simulink model "ZSM_TeslaModelS_statKreisfahrt"  (R2020b)
settings: Solver=FixedStepDiscrete  StartTime=0.0  StopTime=simtime  FixedStep=stepsize  RelTol=1e-3
undefined symbols (not defined in the file): activate_stop, activate_stop_vmax, ay_stop, ayObs, ayStiff, Bat_param, deltav_ist, DiscIntNeverNeededParam, EG_wunsch, magnitude, mu_road_LF, mu_road_LR, mu_road_RF, mu_road_RR, par_ASR, par_MDT, par_TIR, par_VEH, select_delta_h, select_M_wheel, stepsize, t, temp_betriebsstrategie, temperature_LTrange, track_left, track_right
libraries: Library_ASK x36, simulink x16, pid_lib x2, dspstat3 x2, Library_Betriebsstrategie x2, vehicle_model x2, pacejka_trans x1
(part 2 of 7)

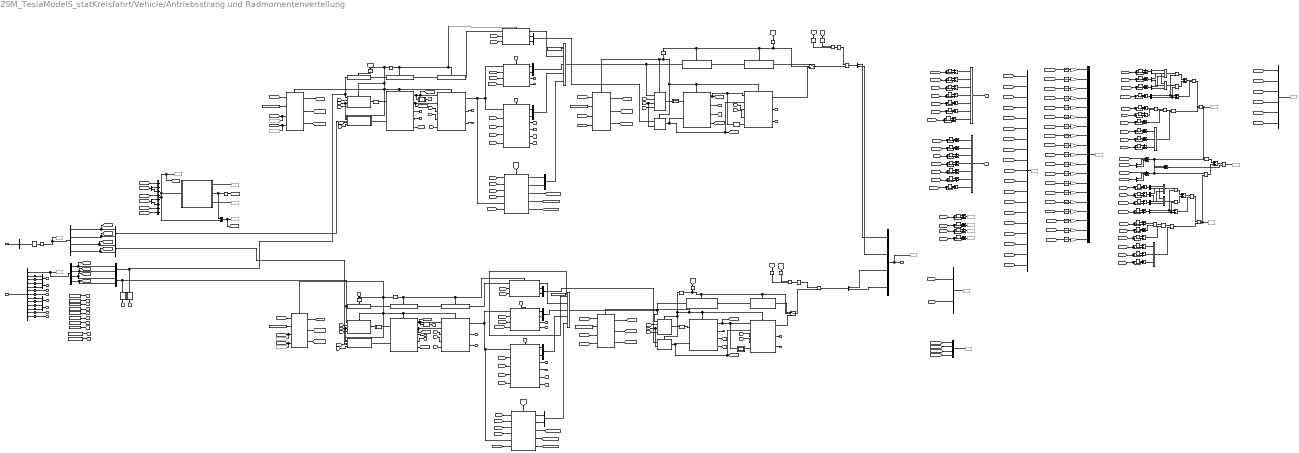
== system ZSM_TeslaModelS_statKreisfahrt/Vehicle/Antriebsstrang und Radmomentenverteilung ==
  note: Rekuperationsindex
  note: Rad-Wunsch-Momente
  note: Rad-Ist-Drehzahlen
  note: Vorderachse
  note: Hinterachse
  note: Overall efficiency of front and rear axle
  note: Gesamtwirkungsgrad des Antriebsstrangs EXKLUSIVE (ausgegraut) und INKLUSIVE (wenn nicht ausgegraut) E-Motor
  note: Verlustenergie
  note: Leistungsaufnahme der E-Maschinen
  note: Verlustleistungen
  note: einzelne Wirkungsgrade
  Ergebnisse der Betriebsstrategie : Inport
  Ergebnisse aus dem Fahrzeugmodell : Inport  Port=2
  Abs1 : Abs
  Add{,1..16,18..42,45..46} (44 alike) : Sum
  Add17 : Sum  Inputs=++++++++
  Add43 : Sum  Inputs=+++
  Add44 : Sum  Inputs=+++
  Batterie : Subsystem
  Bus Creator : BusCreator  Inputs=4
  Bus Creator1 : BusCreator  Inputs=2
  Bus Creator2 : BusCreator  Inputs=19
  Bus Creator3 : BusCreator  Inputs=19
  Bus Creator4 : BusCreator  Inputs=6
  Bus Creator5 : BusCreator  Inputs=4
  Bus Selector : BusSelector  OutputSignals=M_antr,Schaltstrategie.Übersetzungen.i_LF,Schaltstrategie.Übersetzungen.i_RF,Schaltstrategie.Übersetzungen.i_LR,Schaltstrategie.Übersetzungen.i_RR,Schaltstrategie.Übersetzungen.i_F,Schaltstrategie.Übersetzungen.i_R,Schaltstrategie.Wirkungsgrade.eta_LF,Schaltstrategie.Wirkungsgrade.eta_RF,Schaltstrategie.Wirkungsgrade.eta_LR,Schaltstrategie.Wirkungsgrade.eta_RR,Schaltstrategie.Wirkungsgrade.eta_F,Schaltstrategie.Wirkungsgrade.eta_R
  Bus Selector1 : BusSelector  OutputSignals=omega
  Bus to Vector2 : BusToVector
  Constant1 : Constant  Value=par_MDT.AUS.akt.az_VA
  Constant11 : Constant  Value=par_MDT.HA.em.U_RMS
  Constant12 : Constant  Value=par_MDT.HA.em.U_RMS
  Constant13 : Constant  Value=par_MDT.VA.em.U_RMS
  Constant14 : Constant  Value=par_MDT.AUS.akt.TS_VA
  Constant15 : Constant  Value=par_MDT.AUS.akt.TS_HA
  Constant2 : Constant  Value=par_MDT.AUS.akt.az_HA
  Constant22 : Constant  Value=par_MDT.AUS.switch.MVS_HA
  Constant24 : Constant  Value=par_MDT.AUS.switch.MVS_VA
  Constant3 : Constant  Value=par_MDT.AUS.akt.OD_VA
  Constant4 : Constant  Value=par_MDT.AUS.akt.OD_HA
  Constant5 : Constant  Value=par_MDT.AUS.akt.eTV_VA
  Constant6 : Constant  Value=par_MDT.AUS.akt.eTV_HA
  Constant7 : Constant  Value=par_MDT.AUS.akt.rn_VA
  Constant8 : Constant  Value=par_MDT.AUS.akt.rn_HA
  Constant9 : Constant  Value=par_MDT.HA.em.U_RMS
  Demux : Demux
  Demux{1..2,4..15} (14 alike) : Demux  Outputs=2
  Demux3 : Demux
  Discrete-Time Integrator{,1..18} (19 alike) : DiscreteIntegrator  SampleTime=stepsize  ICPrevOutput=DiscIntNeverNeededParam  ICPrevScaledInput=DiscIntNeverNeededParam
  Divide : Product  Inputs=*/
  Divide1 : Product  Inputs=*/
  Divide2 : Product  Inputs=*/
  Drehzahlrückführung az HA : Subsystem
  Drehzahlrückführung az VA : Subsystem
  Drehzahlrückführung rn HA fuer mmG : Library_ASK/Drehzahlrückführung rn fuer mmG  SystemSampleTime=-1  VariantActivationTime=update diagram  Latency=0  AutoFrameSizeCalculation=off
  Drehzahlrückführung rn VA fuer mmG : Library_ASK/Drehzahlrückführung rn fuer mmG  SystemSampleTime=-1  VariantActivationTime=update diagram  Latency=0  AutoFrameSizeCalculation=off
  Elektrisches Überlagerungsgetriebe HA : Library_ASK/Elektrisches Überlagerungsgetriebe HA  SystemSampleTime=-1  VariantActivationTime=update diagram  Latency=0  AutoFrameSizeCalculation=off
      link override Constant: Value=par_MDT.HA.trans.etv.i.i12_I
      link override Constant1: Value=par_MDT.HA.trans.etv.eta.eta12_III
      link override Constant10: Value=par_MDT.HA.trans.etv.eta.etaVTV_34
      link override Constant12: Value=par_MDT.HA.trans.etv.eta.eta12_I
      link override Constant13: Value=par_MDT.HA.trans.etv.eta.eta12_II
      link override Constant2: Value=par_MDT.HA.trans.etv.i.i12_II
      link override Constant3: Value=par_MDT.HA.trans.etv.i.i12_III
      link override Constant4: Value=par_MDT.HA.trans.etv.i.i12_IV
      link override Constant5: Value=par_MDT.HA.trans.etv.M_max_Steuer
      link override Constant6: Value=par_MDT.HA.trans.etv.i.iVTV_1
      link override Constant7: Value=par_MDT.HA.trans.etv.i.iVTV_2
      link override Constant8: Value=par_MDT.HA.trans.etv.eta.eta12_IV
      link override Constant9: Value=par_MDT.HA.trans.etv.eta.etaVTV_12
      link override Momentenkennlinie SEM/M_Antr: BreakpointsForDimension1=par_MDT.HA.trans.etv.Kennfelder.MaxMotorTrqCurve_w  Table=par_MDT.HA.trans.etv.Kennfelder.MaxMotorTrqCurve_M
      link override Momentenkennlinie SEM/M_Reku: BreakpointsForDimension1=par_MDT.HA.trans.etv.Kennfelder.MaxGeneratorTrqCurve_w  Table=par_MDT.HA.trans.etv.Kennfelder.MaxGeneratorTrqCurve_M
      link override eUELG Steuermaschine/Wirkungsgradkennfeld nach Pesce: BreakpointsForDimension1=par_MDT.HA.trans.etv.Kennfelder.MotorEffMap3D_w  BreakpointsForDimension2=par_MDT.HA.trans.etv.Kennfelder.MotorEffMap3D_M  Table=par_MDT.HA.trans.etv.Kennfelder.MotorEffMap3D
  Elektrisches Überlagerungsgetriebe VA : Library_ASK/Elektrisches Überlagerungsgetriebe VA  SystemSampleTime=-1  VariantActivationTime=update diagram  Latency=0  AutoFrameSizeCalculation=off
      link override Constant: Value=par_MDT.VA.trans.etv.i.i12_I
      link override Constant1: Value=par_MDT.VA.trans.etv.eta.eta12_III
      link override Constant10: Value=par_MDT.VA.trans.etv.eta.etaVTV_34
      link override Constant12: Value=par_MDT.VA.trans.etv.eta.eta12_I
      link override Constant13: Value=par_MDT.VA.trans.etv.eta.eta12_II
      link override Constant2: Value=par_MDT.VA.trans.etv.i.i12_II
      link override Constant3: Value=par_MDT.VA.trans.etv.i.i12_III
      link override Constant4: Value=par_MDT.VA.trans.etv.i.i12_IV
      link override Constant5: Value=par_MDT.VA.trans.etv.M_max_Steuer
      link override Constant6: Value=par_MDT.VA.trans.etv.i.iVTV_1
      link override Constant7: Value=par_MDT.VA.trans.etv.i.iVTV_2
      link override Constant8: Value=par_MDT.VA.trans.etv.eta.eta12_IV
      link override Constant9: Value=par_MDT.VA.trans.etv.eta.etaVTV_12
      link override Momentenkennlinie SEM/M_Antr: BreakpointsForDimension1=par_MDT.VA.trans.etv.Kennfelder.MaxMotorTrqCurve_w  Table=par_MDT.VA.trans.etv.Kennfelder.MaxMotorTrqCurve_M
      link override Momentenkennlinie SEM/M_Reku: BreakpointsForDimension1=par_MDT.VA.trans.etv.Kennfelder.MaxGeneratorTrqCurve_w  Table=par_MDT.VA.trans.etv.Kennfelder.MaxGeneratorTrqCurve_M
      link override eUELG Steuermaschine/Wirkungsgradkennfeld nach Pesce: BreakpointsForDimension1=par_MDT.VA.trans.etv.Kennfelder.MotorEffMap3D_w  BreakpointsForDimension2=par_MDT.VA.trans.etv.Kennfelder.MotorEffMap3D_M  Table=par_MDT.VA.trans.etv.Kennfelder.MotorEffMap3D
  HA : Product  Inputs=7
  HA_diff1 : Product  Inputs=3
  Kein Getriebe{,1..3} (4 alike) : Library_ASK/Kein Getriebe  SystemSampleTime=-1  VariantActivationTime=update diagram  Latency=0  AutoFrameSizeCalculation=off
  Kein MVS : Library_ASK/Kein MVS  SystemSampleTime=-1  VariantActivationTime=update diagram  Latency=0  AutoFrameSizeCalculation=off
  Kein MVS1 : Library_ASK/Kein MVS  SystemSampleTime=-1  VariantActivationTime=update diagram  Latency=0  AutoFrameSizeCalculation=off
  Keine E-Maschine : Library_ASK/Keine E-Maschine  SystemSampleTime=-1  VariantActivationTime=update diagram  Latency=0  AutoFrameSizeCalculation=off
  Keine E-Maschine radnah : Library_ASK/Keine E-Maschine  SystemSampleTime=-1  VariantActivationTime=update diagram  Latency=0  AutoFrameSizeCalculation=off
  Keine E-Maschine radnah1 : Library_ASK/Keine E-Maschine  SystemSampleTime=-1  VariantActivationTime=update diagram  Latency=0  AutoFrameSizeCalculation=off
  Keine E-Maschine1 : Library_ASK/Keine E-Maschine  SystemSampleTime=-1  VariantActivationTime=update diagram  Latency=0  AutoFrameSizeCalculation=off
  Keine Rückführung : Library_ASK/Keine Rückführung  SystemSampleTime=-1  VariantActivationTime=update diagram  Latency=0  AutoFrameSizeCalculation=off
  Keine Rückführung1 : Library_ASK/Keine Rückführung  SystemSampleTime=-1  VariantActivationTime=update diagram  Latency=0  AutoFrameSizeCalculation=off
  LF : Product  Inputs=3
  LF1 : Product  Inputs=3
  Leistungselektronik AZ HA : Library_ASK/Leistungselektronik  Efficiency_Map=par_MDT.HA.inv.efficiency_map.efficiency_map_LE  Current=par_MDT.HA.inv.current  Voltage=par_MDT.HA.inv.voltage  Powerfactor=par_MDT.HA.inv.powerfactor  Powerfactor_Map=par_MDT.HA.inv.Powerfactor_map  Torque=par_MDT.HA.inv.torque  Speed=par_MDT.HA.inv.speed
  Leistungselektronik AZ VA : Library_ASK/Leistungselektronik  Efficiency_Map=par_MDT.VA.inv.efficiency_map.efficiency_map_LE  Current=par_MDT.VA.inv.current  Voltage=par_MDT.VA.inv.voltage  Powerfactor=par_MDT.VA.inv.powerfactor  Powerfactor_Map=par_MDT.VA.inv.Powerfactor_map  Torque=par_MDT.VA.inv.torque  Speed=par_MDT.VA.inv.speed
  Leistungselektronik RN HA : Library_ASK/Leistungselektronik  Efficiency_Map=par_MDT.HA.inv.efficiency_map.efficiency_map_LE  Current=par_MDT.HA.inv.current  Voltage=par_MDT.HA.inv.voltage  Powerfactor=par_MDT.HA.inv.powerfactor  Powerfactor_Map=par_MDT.HA.inv.Powerfactor_map  Torque=par_MDT.HA.inv.torque  Speed=par_MDT.HA.inv.speed
  Leistungselektronik RN VA : Library_ASK/Leistungselektronik  Efficiency_Map=par_MDT.VA.inv.efficiency_map.efficiency_map_LE  Current=par_MDT.VA.inv.current  Voltage=par_MDT.VA.inv.voltage  Powerfactor=par_MDT.VA.inv.powerfactor  Powerfactor_Map=par_MDT.VA.inv.Powerfactor_map  Torque=par_MDT.VA.inv.torque  Speed=par_MDT.VA.inv.speed
  Logical Operator{,1..15,32..53} (38 alike) : Logic  Operator=NOT  Inputs=1  AllPortsSameDT=off  OutDataTypeStr=boolean
  Logical Operator{16..24,26..28,30..31} (14 alike) : Logic  Operator=NOT  AllPortsSameDT=off  OutDataTypeStr=boolean
  Logical Operator25 : Logic  AllPortsSameDT=off  OutDataTypeStr=boolean
  Logical Operator29 : Logic  AllPortsSameDT=off  OutDataTypeStr=boolean
  MATLAB Function : MATLAB Function  TreatAsAtomicUnit=on
  MATLAB Function1 : MATLAB Function  TreatAsAtomicUnit=on
  MATLAB Function2 : MATLAB Function  TreatAsAtomicUnit=on
  MATLAB Function3 : MATLAB Function  TreatAsAtomicUnit=on
  MATLAB Function4 : MATLAB Function  TreatAsAtomicUnit=on
  MATLAB Function5 : MATLAB Function  TreatAsAtomicUnit=on
  Mehrstufiges und mehrgängiges Getriebe az : Library_ASK/Mehrstufiges und mehrgängiges Getriebe  SystemSampleTime=-1  VariantActivationTime=update diagram  Latency=0  AutoFrameSizeCalculation=off
  Mehrstufiges und mehrgängiges Getriebe az1 : Library_ASK/Mehrstufiges und mehrgängiges Getriebe  SystemSampleTime=-1  VariantActivationTime=update diagram  Latency=0  AutoFrameSizeCalculation=off
  Mehrstufiges und mehrgängiges Getriebe rn : Library_ASK/Mehrstufiges und mehrgängiges Getriebe  SystemSampleTime=-1  VariantActivationTime=update diagram  Latency=0  AutoFrameSizeCalculation=off
  Mehrstufiges und mehrgängiges Getriebe rn1 : Library_ASK/Mehrstufiges und mehrgängiges Getriebe  SystemSampleTime=-1  VariantActivationTime=update diagram  Latency=0  AutoFrameSizeCalculation=off
  Memory{,2,6..15} (12 alike) : Memory  InitialCondition=10
  Memory1 : Memory
  Momentenrückführung HA fuer mmG : Library_ASK/Momentenrückführung fuer mmG  SystemSampleTime=-1  VariantActivationTime=update diagram  Latency=0  AutoFrameSizeCalculation=off
  Momentenrückführung HA fuer mmG3 : Library_ASK/Momentenrückführung fuer mmG  SystemSampleTime=-1  VariantActivationTime=update diagram  Latency=0  AutoFrameSizeCalculation=off
  Momentenrückführung VA fuer mmG : Library_ASK/Momentenrückführung fuer mmG  SystemSampleTime=-1  VariantActivationTime=update diagram  Latency=0  AutoFrameSizeCalculation=off
  Momentenrückführung VA fuer mmG1 : Library_ASK/Momentenrückführung fuer mmG  SystemSampleTime=-1  VariantActivationTime=update diagram  Latency=0  AutoFrameSizeCalculation=off
  Multiport Switch1 : MultiPortSwitch  Inputs=4
  Multiport Switch2 : MultiPortSwitch  Inputs=4
  Mux{,1..9,15..18,22..23} (16 alike) : Mux  Inputs=2
  Offenes Differential HA : Library_ASK/Offenes Differential  M_max=par_MDT.HA.em.M_max_achse  i_max=par_MDT.HA.trans.imax
      link override Constant2: Value=par_MDT.AUS.eta_Kegel
  Offenes Differential VA : Library_ASK/Offenes Differential  M_max=par_MDT.VA.em.M_max_achse  i_max=par_MDT.VA.trans.imax
      link override Constant2: Value=par_MDT.AUS.eta_Kegel
  PT_HA1 : Subsystem
  PT_HA2 : Subsystem
  PT_VA : Subsystem
  PT_VA1 : Subsystem
  Product{1..14} (14 alike) : Product
  RF : Product  Inputs=3
  RF1 : Product  Inputs=3
  Simple E-Maschine HA : Library_ASK/Simple E-Maschine  Mot_Mmax_Curve=par_MDT.HA.em.MaxMotorTrqCurve_M  Mot_nmax_Curve=par_MDT.HA.em.MaxMotorTrqCurve_w  Gen_Mmax_Curve=par_MDT.HA.em.MaxGeneratorTrqCurve_M  Gen_nmax_Curve=par_MDT.HA.em.MaxGeneratorTrqCurve_w  Mot_Pesce_Mat=par_MDT.HA.em.MotorEffMap3D  Mot_Pesce_y=par_MDT.HA.em.MotorEffMap3D_w  Mot_Pesce_z=par_MDT.HA.em.MotorEffMap3D_M  Gen_Pesce_Mat=par_MDT.HA.em.GeneratorEffMap3D  Gen_Pesce_y=par_MDT.HA.em.GeneratorEffMap3D_w  Gen_Pesce_z=par_MDT.HA.em.GeneratorEffMap3D_M
  Simple E-Maschine VA : Library_ASK/Simple E-Maschine  Mot_Mmax_Curve=par_MDT.VA.em.MaxMotorTrqCurve_M  Mot_nmax_Curve=par_MDT.VA.em.MaxMotorTrqCurve_w  Gen_Mmax_Curve=par_MDT.VA.em.MaxGeneratorTrqCurve_M  Gen_nmax_Curve=par_MDT.VA.em.MaxGeneratorTrqCurve_w  Mot_Pesce_Mat=par_MDT.VA.em.MotorEffMap3D  Mot_Pesce_y=par_MDT.VA.em.MotorEffMap3D_w  Mot_Pesce_z=par_MDT.VA.em.MotorEffMap3D_M  Gen_Pesce_Mat=par_MDT.VA.em.GeneratorEffMap3D  Gen_Pesce_y=par_MDT.VA.em.GeneratorEffMap3D_w  Gen_Pesce_z=par_MDT.VA.em.GeneratorEffMap3D_M
  Simple E-Maschine radnah : Library_ASK/Simple E-Maschine radnah  Mot_Mmax_Curve=par_MDT.VA.em.MaxMotorTrqCurve_M  Mot_nmax_Curve=par_MDT.VA.em.MaxMotorTrqCurve_w  Gen_Mmax_Curve=par_MDT.VA.em.MaxGeneratorTrqCurve_M  Gen_nmax_Curve=par_MDT.VA.em.MaxGeneratorTrqCurve_w  Mot_Pesce_Mat=par_MDT.VA.em.MotorEffMap3D  Mot_Pesce_y=par_MDT.VA.em.MotorEffMap3D_w  Mot_Pesce_z=par_MDT.VA.em.MotorEffMap3D_M  Gen_Pesce_Mat=par_MDT.VA.em.GeneratorEffMap3D  Gen_Pesce_y=par_MDT.VA.em.GeneratorEffMap3D_w  Gen_Pesce_z=par_MDT.VA.em.GeneratorEffMap3D_M
  Simple E-Maschine radnah1 : Library_ASK/Simple E-Maschine radnah  Mot_Mmax_Curve=par_MDT.HA.em.MaxMotorTrqCurve_M  Mot_nmax_Curve=par_MDT.HA.em.MaxMotorTrqCurve_w  Gen_Mmax_Curve=par_MDT.HA.em.MaxGeneratorTrqCurve_M  Gen_nmax_Curve=par_MDT.HA.em.MaxGeneratorTrqCurve_w  Mot_Pesce_Mat=par_MDT.HA.em.MotorEffMap3D  Mot_Pesce_y=par_MDT.HA.em.MotorEffMap3D_w  Mot_Pesce_z=par_MDT.HA.em.MotorEffMap3D_M  Gen_Pesce_Mat=par_MDT.HA.em.GeneratorEffMap3D  Gen_Pesce_y=par_MDT.HA.em.GeneratorEffMap3D_w  Gen_Pesce_z=par_MDT.HA.em.GeneratorEffMap3D_M
  Sum1 : Sum
  Switch1 : Switch  Criteria=u2 > Threshold
  Switch3 : Switch  Criteria=u2 > Threshold
  To Workspace : ToWorkspace  Commented=on  VariableName=n_Rad_ist  SampleTime=-1
      settings: Decimation=savedec  Save2DSignal=2-D array (concatenate along first dimension)
  To Workspace11 : ToWorkspace  Commented=on  VariableName=Batt_SOC  SaveFormat=Timeseries  SampleTime=-1
  To Workspace12 : ToWorkspace  Commented=on  VariableName=Batt_C_Rate  SaveFormat=Timeseries  SampleTime=-1
  To Workspace20 : ToWorkspace  Commented=on  VariableName=eta_ges  SaveFormat=Timeseries  SampleTime=-1
      settings: Decimation=savedec
  To Workspace3 : ToWorkspace  Commented=on  VariableName=P_Batt  SaveFormat=Timeseries  SampleTime=-1
  To Workspace4 : ToWorkspace  Commented=on  VariableName=M_antr  SaveFormat=Timeseries  SampleTime=-1
  To Workspace5 : ToWorkspace  Commented=on  VariableName=M_Rad_W  SampleTime=-1
      settings: Decimation=savedec  Save2DSignal=2-D array (concatenate along first dimension)
  To Workspace9 : ToWorkspace  Commented=on  VariableName=P_LE_DC  SaveFormat=Timeseries  SampleTime=-1
  To Ws 1 : ToWorkspace  Commented=on  VariableName=pv_ges  SaveFormat=Timeseries  SampleTime=-1
      settings: Decimation=savedec  Save2DSignal=2-D array (concatenate along first dimension)
  To Ws 10 : ToWorkspace  Commented=on  VariableName=eta_EM_rn_HA  SaveFormat=Timeseries  SampleTime=-1
      settings: Decimation=savedec  Save2DSignal=2-D array (concatenate along first dimension)
  To Ws 11 : ToWorkspace  Commented=on  VariableName=eta_LE  SaveFormat=Timeseries  SampleTime=-1
      settings: Decimation=savedec  Save2DSignal=2-D array (concatenate along first dimension)
  To Ws 12 : ToWorkspace  Commented=on  VariableName=eta_AS_ges  SaveFormat=Timeseries  SampleTime=-1
      settings: Decimation=savedec  Save2DSignal=2-D array (concatenate along first dimension)
  To Ws 14 : ToWorkspace  Commented=on  VariableName=sv_n_mot_az_ha  SaveFormat=Timeseries  SampleTime=-1
      settings: Decimation=savedec  Save2DSignal=2-D array (concatenate along first dimension)
  To Ws 15 : ToWorkspace  Commented=on  VariableName=sv_n_mot_az_va  SaveFormat=Timeseries  SampleTime=-1
      settings: Decimation=savedec  Save2DSignal=2-D array (concatenate along first dimension)
  To Ws 2 : ToWorkspace  Commented=on  VariableName=sv_m_mot_az_va  SaveFormat=Timeseries  SampleTime=-1
      settings: Decimation=savedec  Save2DSignal=2-D array (concatenate along first dimension)
  To Ws 3 : ToWorkspace  Commented=on  VariableName=eta_VA  SaveFormat=Timeseries  SampleTime=-1
      settings: Decimation=savedec  Save2DSignal=2-D array (concatenate along first dimension)
  To Ws 4 : ToWorkspace  Commented=on  VariableName=eta_HA  SaveFormat=Timeseries  SampleTime=-1
      settings: Decimation=savedec  Save2DSignal=2-D array (concatenate along first dimension)
  To Ws 5 : ToWorkspace  Commented=on  VariableName=Ev_ges  SaveFormat=Timeseries  SampleTime=-1
      settings: Decimation=savedec  Save2DSignal=2-D array (concatenate along first dimension)
  To Ws 6 : ToWorkspace  Commented=on  VariableName=P_el  SaveFormat=Timeseries  SampleTime=-1
      settings: Decimation=savedec  Save2DSignal=2-D array (concatenate along first dimension)
  To Ws 7 : ToWorkspace  Commented=on  VariableName=eta_EM_az_VA  SaveFormat=Timeseries  SampleTime=-1
      settings: Decimation=savedec  Save2DSignal=2-D array (concatenate along first dimension)
  To Ws 8 : ToWorkspace  Commented=on  VariableName=eta_EM_rn_VA  SaveFormat=Timeseries  SampleTime=-1
      settings: Decimation=savedec  Save2DSignal=2-D array (concatenate along first dimension)
  To Ws 9 : ToWorkspace  Commented=on  VariableName=eta_EM_az_HA  SaveFormat=Timeseries  SampleTime=-1
      settings: Decimation=savedec  Save2DSignal=2-D array (concatenate along first dimension)
  "To Ws 13 " : ToWorkspace  Commented=on  VariableName=sv_m_mot_az_ha  SaveFormat=Timeseries  SampleTime=-1
      settings: Decimation=savedec  Save2DSignal=2-D array (concatenate along first dimension)
  Torque Splitter v2 C. Angerer 10/1 : Library_ASK/Torque Splitter v2 C. Angerer 10//2018  SystemSampleTime=-1  VariantActivationTime=update diagram  Latency=0  AutoFrameSizeCalculation=off
  Torque Splitter v2 C. Angerer 10/2018 : Library_ASK/Torque Splitter v2 C. Angerer 10//2018  SystemSampleTime=-1  VariantActivationTime=update diagram  Latency=0  AutoFrameSizeCalculation=off
  VA : Product  Inputs=7
  VA_diff : Product  Inputs=3
  kWs --> kWh{,1..18} (19 alike) : Gain  Gain=1/3600
  w/o E-maschine HA : Product  Inputs=**
  w/o E-maschine VA : Product  Inputs=**
  M_antr : Outport  VectorParamsAs1DForOutWhenUnconnected=off
  wires:
  Bus Selector1/1 -> Bus to Vector2/1  "<omega>"
  Ergebnisse aus dem Fahrzeugmodell/1 -> Bus Selector1/1
  [OD_VA] -> Offenes Differential VA/Enable
  Mux/1 -> Keine Rückführung/1, Momentenrückführung VA fuer mmG/1, MATLAB Function/1(u)
  Demux/1 -> Mux/1, [M_Rad_W_RF]  "M_Rad_W_RF"
  Demux/2 -> Mux/2, [M_Rad_W_LF]  "M_Rad_W_LF"
  Logical Operator16/1 -> Kein MVS/Enable, Kein Getriebe/Enable, Keine E-Maschine/Enable
  Kein MVS/1 -> Multiport Switch1/2  "2"
  Demux/4 -> [M_Rad_W_LR], Mux1/2  "M_Rad_W_LR"
  Demux/3 -> Mux1/1, [M_Rad_W_RR]  "M_Rad_W_RR"
  Bus Creator/1 -> To Workspace4/1, M_antr/1
  Offenes Differential VA/2 -> Mux2/2  "1"
  Offenes Differential VA/1 -> Mux2/1  "1"
  Elektrisches Überlagerungsgetriebe VA/2 -> Mux3/2
  Elektrisches Überlagerungsgetriebe VA/1 -> Mux3/1
  Mux2/1 -> Multiport Switch1/3  "2"
  Demux1/1 -> Bus Creator/1  "M_antr_RF"
  Demux1/2 -> Bus Creator/2  "M_antr_LF"
  Kein Getriebe2/1 -> Switch3/1
  Constant24/1 -> Multiport Switch1/1
  [n_Rad_RF] -> Kein MVS/2
  [n_Rad_LF] -> Kein MVS/3
  Kein Getriebe/1 -> Kein MVS/1
  Mux15/1 -> Drehzahlrückführung az VA/3("Radrehzahlen ")
  Simple E-Maschine VA/3 -> [pv_simEM_az_VA]
  Kein MVS/2 -> Mux8/1
  Kein MVS/3 -> Mux8/2
  Demux3/1 -> Mux15/1, [n_Rad_RF]
  Demux3/2 -> Mux15/2, [n_Rad_LF]
  Demux3/3 -> Mux16/1, [n_Rad_RR]
  Demux3/4 -> [n_Rad_LR], Mux16/2
  Memory1/1 -> To Workspace/1, Demux3/1  "n_Rad_ist"
  Momentenrückführung VA fuer mmG/1 -> PT_VA1/1(M)
  Keine E-Maschine/1 -> Kein Getriebe/1
  Mux3/1 -> Multiport Switch1/4
  Multiport Switch1/1 -> Momentenrückführung VA fuer mmG1/1, Keine E-Maschine radnah/1  "2"
  Mux8/1 -> Drehzahlrückführung rn VA fuer mmG/1
  Keine E-Maschine radnah/1 -> Kein Getriebe2/1
  Demux2/1 -> Bus Creator/3  "M_antr_RR"
  Demux2/2 -> Bus Creator/4  "M_antr_LR"
  Bus to Vector2/1 -> Memory1/1
  Ergebnisse der Betriebsstrategie/1 -> Bus Selector/1
  Bus Selector/1 -> To Workspace5/1, Demux/1  "<M_antr>"
  [n_Rad_LF] -> Offenes Differential VA/3
  [n_Rad_RF] -> Elektrisches Überlagerungsgetriebe VA/2
  [n_Rad_LF] -> Elektrisches Überlagerungsgetriebe VA/3
  [M_Rad_W_RF] -> Elektrisches Überlagerungsgetriebe VA/4
  [M_Rad_W_LF] -> Elektrisches Überlagerungsgetriebe VA/5
  [n_Rad_RF] -> Offenes Differential VA/2
  [az_VA] -> Logical Operator16/1, Momentenrückführung VA fuer mmG/Enable, Mehrstufiges und mehrgängiges Getriebe az/Enable, Simple E-Maschine VA/Enable, Leistungselektronik AZ VA/Enable, Drehzahlrückführung az VA/1(Aktivator az), Logical Operator17/1
  Mehrstufiges und mehrgängiges Getriebe rn/1 -> Switch3/3
  [rn_VA] -> Logical Operator22/1
  [eta_VA] -> Momentenrückführung VA fuer mmG1/2
  [i_Gang_az_VA] -> Drehzahlrückführung az VA/2("i_Gang "), Momentenrückführung VA fuer mmG/3
  Keine Rückführung/1 -> Keine E-Maschine/1
  Mux17/1 -> [i_Gang_rn_VA]
  Mux18/1 -> [i_Gang_rn_HA]
  Mux22/1 -> [eta_Gang_rn_VA]
  Mux23/1 -> [eta_Gang_rn_HA]
  [i_Gang_rn_VA] -> Momentenrückführung VA fuer mmG1/3, Drehzahlrückführung rn VA fuer mmG/2
  [OD_HA] -> Offenes Differential HA/Enable
  [eTV_HA] -> Elektrisches Überlagerungsgetriebe HA/Enable
  Logical Operator20/1 -> Kein MVS1/Enable, Kein Getriebe1/Enable, Keine E-Maschine1/Enable
  Kein MVS1/1 -> Multiport Switch2/2  "2"
  Offenes Differential HA/2 -> Mux4/2  "1"
  Offenes Differential HA/1 -> Mux4/1  "1"
  Elektrisches Überlagerungsgetriebe HA/2 -> Mux5/2
  Elektrisches Überlagerungsgetriebe HA/1 -> Mux5/1
  Mux4/1 -> Multiport Switch2/3  "2"
  Kein Getriebe3/1 -> Switch1/1
  [rn_HA] -> Logical Operator26/1
  Constant22/1 -> Multiport Switch2/1
  [n_Rad_RR] -> Kein MVS1/2
  [n_Rad_LR] -> Kein MVS1/3
  Kein Getriebe1/1 -> Kein MVS1/1
  Kein MVS1/2 -> Mux6/1
  Kein MVS1/3 -> Mux6/2
  Momentenrückführung HA fuer mmG/1 -> PT_HA1/1(M)
  Keine E-Maschine1/1 -> Kein Getriebe1/1
  Mux5/1 -> Multiport Switch2/4
  Momentenrückführung HA fuer mmG3/1 -> PT_HA2/1(M)
  Multiport Switch2/1 -> Keine E-Maschine radnah1/1, Momentenrückführung HA fuer mmG3/1  "2"
  Mux6/1 -> Drehzahlrückführung rn HA fuer mmG/1
  Drehzahlrückführung rn HA fuer mmG/1 -> Simple E-Maschine radnah1/2, Mehrstufiges und mehrgängiges Getriebe rn1/2, [n_mot_rn_ha]
  Keine E-Maschine radnah1/1 -> Kein Getriebe3/1
  [n_Rad_LR] -> Offenes Differential HA/3
  [n_Rad_RR] -> Elektrisches Überlagerungsgetriebe HA/2
  [n_Rad_LR] -> Elektrisches Überlagerungsgetriebe HA/3
  [M_Rad_W_RR] -> Elektrisches Überlagerungsgetriebe HA/4
  [M_Rad_W_LR] -> Elektrisches Überlagerungsgetriebe HA/5
  Simple E-Maschine radnah1/3 -> [eta_EM_rn_HA]
  [n_Rad_RR] -> Offenes Differential HA/2
  [az_HA] -> Leistungselektronik AZ HA/Enable, Logical Operator20/1, Momentenrückführung HA fuer mmG/Enable, Drehzahlrückführung az HA/1(Aktivator az), Mehrstufiges und mehrgängiges Getriebe az1/Enable, Simple E-Maschine HA/Enable, Logical Operator18/1
  Mehrstufiges und mehrgängiges Getriebe rn1/1 -> Switch1/3
  Mehrstufiges und mehrgängiges Getriebe rn1/3 -> [eta_GTR_rn_HA]
  Logical Operator21/1 -> Leistungselektronik RN HA/Enable, Simple E-Maschine radnah1/Enable, Mehrstufiges und mehrgängiges Getriebe rn1/Enable, Drehzahlrückführung rn HA fuer mmG/Enable, Momentenrückführung HA fuer mmG3/Enable
  [eta_HA] -> Momentenrückführung HA fuer mmG/2
  [eta_HA] -> Momentenrückführung HA fuer mmG3/2
  [i_Gang_az_HA] -> Momentenrückführung HA fuer mmG/3, Drehzahlrückführung az HA/2("i_Gang ")
  Keine Rückführung1/1 -> Keine E-Maschine1/1
  Logical Operator18/1 -> Keine Rückführung1/Enable
  [i_Gang_az_HA] -> Mehrstufiges und mehrgängiges Getriebe az1/3
  [eta_Gang_az_HA] -> Mehrstufiges und mehrgängiges Getriebe az1/4
  [i_Gang_rn_HA] -> Momentenrückführung HA fuer mmG3/3, Drehzahlrückführung rn HA fuer mmG/2
  [i_Gang_rn_HA] -> Mehrstufiges und mehrgängiges Getriebe rn1/3
  [eta_Gang_rn_HA] -> Mehrstufiges und mehrgängiges Getriebe rn1/4
  Mux16/1 -> Drehzahlrückführung az HA/3("Radrehzahlen ")
  Bus Selector/2 -> Memory/1  "<i_LF>"
  Bus Selector/3 -> Memory2/1  "<i_RF>"
  Bus Selector/4 -> Memory6/1  "<i_LR>"
  Bus Selector/5 -> Memory7/1  "<i_RR>"
  Bus Selector/6 -> Memory8/1  "<i_F>"
  Bus Selector/7 -> Memory9/1  "<i_R>"
  Bus Selector/8 -> Memory10/1  "<eta_LF>"
  Bus Selector/9 -> Memory11/1  "<eta_RF>"
  Bus Selector/10 -> Memory12/1  "<eta_LR>"
  Bus Selector/11 -> Memory13/1  "<eta_RR>"
  Bus Selector/12 -> Memory14/1  "<eta_F>"
  Bus Selector/13 -> Memory15/1  "<eta_R>"
  Memory/1 -> Mux17/1
  Memory2/1 -> Mux17/2
  Memory6/1 -> Mux18/1
  Memory7/1 -> Mux18/2
  Memory8/1 -> [i_Gang_az_VA]
  Memory9/1 -> [i_Gang_az_HA]
  Memory10/1 -> Mux22/1
  Memory11/1 -> Mux22/2
  Memory12/1 -> Mux23/1
  Memory13/1 -> Mux23/2
  Memory14/1 -> [eta_Gang_az_VA]
  Memory15/1 -> [eta_Gang_az_HA]
  Constant1/1 -> [az_VA]
  Constant2/1 -> [az_HA]
  Constant3/1 -> [OD_VA]
  Constant4/1 -> [OD_HA]
  Constant5/1 -> [eTV_VA]
  Constant6/1 -> [eTV_HA]
  Logical Operator17/1 -> Keine Rückführung/Enable
  Logical Operator19/1 -> Mehrstufiges und mehrgängiges Getriebe rn/Enable, Simple E-Maschine radnah/Enable, Drehzahlrückführung rn VA fuer mmG/Enable, Leistungselektronik RN VA/Enable, Momentenrückführung VA fuer mmG1/Enable
  MATLAB Function1/1(RIX) -> [RIX_HA]
  MATLAB Function/1(RIX) -> [RIX_VA]
  [RIX_VA] -> Momentenrückführung VA fuer mmG/4
  [RIX_HA] -> Momentenrückführung HA fuer mmG/4
  [RIX_VA] -> Momentenrückführung VA fuer mmG1/4
  [RIX_HA] -> Momentenrückführung HA fuer mmG3/4
  Elektrisches Überlagerungsgetriebe VA/3 -> [pv_ges_eUELG_VA]
  Elektrisches Überlagerungsgetriebe VA/4 -> [M_Steuer_eUELG_VA]
  Elektrisches Überlagerungsgetriebe VA/5 -> [eta_eUELG_VA]
  Elektrisches Überlagerungsgetriebe VA/6 -> [P_Batt_eUELG_VA]
  Elektrisches Überlagerungsgetriebe HA/6 -> [P_Batt_eUELG_HA]
  Elektrisches Überlagerungsgetriebe HA/5 -> [eta_eUELG_HA]
  Elektrisches Überlagerungsgetriebe HA/4 -> [M_Steuer_eUELG_HA]
  Elektrisches Überlagerungsgetriebe HA/3 -> [pv_ges_eUELG_HA]
  Simple E-Maschine VA/4 -> [eta_EM_az_VA]
  Mehrstufiges und mehrgängiges Getriebe az/3 -> [eta_GTR_az_VA]
  Mehrstufiges und mehrgängiges Getriebe az/2 -> [pv_GTR_az_VA]
  Offenes Differential VA/4 -> [eta_OD_VA]
  Offenes Differential VA/3 -> [pv_OD_VA]
  Simple E-Maschine radnah/2 -> [pv_simEM_rn_VA]
  Simple E-Maschine radnah/3 -> [eta_EM_rn_VA]
  Mehrstufiges und mehrgängiges Getriebe rn/2 -> [pv_GTR_rn_VA]
  Mehrstufiges und mehrgängiges Getriebe rn/3 -> [eta_GTR_rn_VA]
  Simple E-Maschine HA/3 -> [pv_simEM_az_HA]
  Simple E-Maschine HA/4 -> [eta_EM_az_HA]
  Mehrstufiges und mehrgängiges Getriebe az1/2 -> [pv_GTR_az_HA]
  Mehrstufiges und mehrgängiges Getriebe az1/3 -> [eta_GTR_az_HA]
  Simple E-Maschine radnah1/2 -> [pv_simEM_rn_HA]
  Mehrstufiges und mehrgängiges Getriebe rn1/2 -> [pv_GTR_rn_HA]
  [RIX_VA_Delayed] -> Offenes Differential VA/4
  Offenes Differential HA/3 -> [pv_OD_HA]
  Offenes Differential HA/4 -> [eta_OD_HA]
  [RIX_VA_Delayed] -> Mehrstufiges und mehrgängiges Getriebe az/5
  [eta_Gang_az_VA] -> Mehrstufiges und mehrgängiges Getriebe az/4
  [i_Gang_az_VA] -> Mehrstufiges und mehrgängiges Getriebe az/3
  [i_Gang_rn_VA] -> Mehrstufiges und mehrgängiges Getriebe rn/3
  [eta_Gang_rn_VA] -> Mehrstufiges und mehrgängiges Getriebe rn/4
  MATLAB Function3/1(RIX) -> Mehrstufiges und mehrgängiges Getriebe rn/5
  Simple E-Maschine HA/2 -> [n_mot_az_ha], Mehrstufiges und mehrgängiges Getriebe az1/2
  [RIX_HA_Delayed] -> Mehrstufiges und mehrgängiges Getriebe az1/5
  Momentenrückführung VA fuer mmG1/1 -> PT_VA/1(M)  "2"
  [eta_VA] -> Momentenrückführung VA fuer mmG/2
  PT_VA/1(M_d) -> Simple E-Maschine radnah/1
  PT_VA1/1(M_d) -> Simple E-Maschine VA/1
  PT_HA1/1(M_d) -> Simple E-Maschine HA/1
  PT_HA2/1(M_d) -> Simple E-Maschine radnah1/1
  Simple E-Maschine VA/5 -> [P_el_EM_az_VA]
  Simple E-Maschine radnah/4 -> [P_el_EM_rn_VA]
  Simple E-Maschine radnah1/4 -> [P_el_EM_rn_HA]
  Simple E-Maschine HA/5 -> [P_el_EM_az_HA]
  Constant8/1 -> [rn_HA]
  Constant7/1 -> [rn_VA]
  Logical Operator22/1 -> Logical Operator19/1, Keine E-Maschine radnah/Enable, Kein Getriebe2/Enable, Switch3/2
  [rn_VA] -> Logical Operator24/1
  [az_VA] -> Logical Operator23/1
  Logical Operator23/1 -> Logical Operator25/2
  Logical Operator24/1 -> Logical Operator25/1
  Switch3/1 -> w/o E-maschine VA/2
  w/o E-maschine VA/1 -> Demux1/1
  Logical Operator26/1 -> Switch1/2, Kein Getriebe3/Enable, Keine E-Maschine radnah1/Enable, Logical Operator21/1
  Logical Operator27/1 -> Logical Operator29/2
  Logical Operator28/1 -> Logical Operator29/1
  [rn_HA] -> Logical Operator28/1
  [az_HA] -> Logical Operator27/1
  Switch1/1 -> w/o E-maschine HA/2
  w/o E-maschine HA/1 -> Demux2/1
  Logical Operator29/1 -> Logical Operator30/1
  Logical Operator30/1 -> w/o E-maschine HA/1
  Logical Operator25/1 -> Logical Operator31/1
  Logical Operator31/1 -> w/o E-maschine VA/1
  [P_LE_DC_HA_RN] -> Demux6/1
  [P_LE_DC_VA_AZ] -> Add17/1
  Demux6/2 -> Add17/6
  Batterie/3(C-Rate) -> To Workspace12/1
  Add17/1 -> Batterie/1(P_LE_DC), [P_LE_DC], To Workspace9/1, Sum1/2
  Sum1/1 -> [P_Batt], To Workspace3/1
  Batterie/2(pv_batt) -> Sum1/1, Abs1/1
  Demux5/2 -> Add17/3
  Demux5/1 -> Add17/2
  Batterie/1(SOC) -> To Workspace11/1
  Abs1/1 -> [pv_Batt]
  [P_LE_DC_HA_AZ] -> Add17/4
  Demux6/1 -> Add17/5
  [P_LE_DC_VA_RN] -> Demux5/1
  [P_el_EM_rn_VA] -> Leistungselektronik RN VA/1
  Constant9/1 -> Leistungselektronik RN VA/2
  [m_mot_rn_va] -> Leistungselektronik RN VA/3
  [n_mot_rn_va] -> Leistungselektronik RN VA/4
  [P_el_EM_rn_HA] -> Leistungselektronik RN HA/1
  Constant11/1 -> Leistungselektronik RN HA/2
  [m_mot_rn_ha] -> Leistungselektronik RN HA/3
  [n_mot_rn_ha] -> Leistungselektronik RN HA/4
  [P_el_EM_az_HA] -> Leistungselektronik AZ HA/1
  Constant12/1 -> Leistungselektronik AZ HA/2
  [m_mot_az_ha] -> "To Ws 13 "/1, Leistungselektronik AZ HA/3
  [n_mot_az_ha] -> To Ws 14/1, Leistungselektronik AZ HA/4
  [P_el_EM_az_VA] -> Leistungselektronik AZ VA/1
  Constant13/1 -> Leistungselektronik AZ VA/2
  [m_mot_az_va] -> To Ws 2/1, Leistungselektronik AZ VA/3
  [n_mot_az_va] -> To Ws 15/1, Leistungselektronik AZ VA/4
  Leistungselektronik AZ VA/1 -> [eta_LE_VA_AZ]
  Leistungselektronik AZ VA/2 -> [pv_LE_VA_AZ]
  Leistungselektronik AZ VA/3 -> [P_LE_DC_VA_AZ]
  Leistungselektronik AZ HA/1 -> [eta_LE_HA_AZ]
  Leistungselektronik AZ HA/2 -> [pv_LE_HA_AZ]
  Leistungselektronik AZ HA/3 -> [P_LE_DC_HA_AZ]
  Leistungselektronik RN HA/1 -> [eta_LE_HA_RN]
  Leistungselektronik RN HA/2 -> [pv_LE_HA_RN]
  Leistungselektronik RN HA/3 -> [P_LE_DC_HA_RN]
  Leistungselektronik RN VA/1 -> [eta_LE_VA_RN]
  Leistungselektronik RN VA/2 -> [pv_LE_VA_RN]
  Leistungselektronik RN VA/3 -> [P_LE_DC_VA_RN]
  Mehrstufiges und mehrgängiges Getriebe az1/1 -> Offenes Differential HA/1, Torque Splitter v2 C. Angerer 10/1/5, Elektrisches Überlagerungsgetriebe HA/1
  [TS_HA] -> Torque Splitter v2 C. Angerer 10/1/Enable
  Constant15/1 -> [TS_HA]
  Constant14/1 -> [TS_VA]
  Torque Splitter v2 C. Angerer 10/1/3 -> [n_Kupplung_geschlossen_HA]
  Torque Splitter v2 C. Angerer 10/1/2 -> Mux7/2
  Torque Splitter v2 C. Angerer 10/1/1 -> Mux7/1
  Torque Splitter v2 C. Angerer 10/1/4 -> [p_v_TS_HA]
  Torque Splitter v2 C. Angerer 10/1/5 -> [eta_TS_HA]
  [RIX_HA_Delayed] -> Torque Splitter v2 C. Angerer 10/1/6
  [M_Rad_W_LR] -> Torque Splitter v2 C. Angerer 10/1/4
  [M_Rad_W_RR] -> Torque Splitter v2 C. Angerer 10/1/3
  [n_Rad_LR] -> Torque Splitter v2 C. Angerer 10/1/2
  [n_Rad_RR] -> Torque Splitter v2 C. Angerer 10/1/1
  Mehrstufiges und mehrgängiges Getriebe az/1 -> Torque Splitter v2 C. Angerer 10/2018/5, Offenes Differential VA/1, Elektrisches Überlagerungsgetriebe VA/1
  Mux9/1 -> Multiport Switch1/5
  Torque Splitter v2 C. Angerer 10/2018/5 -> [eta_TS_VA]
  Torque Splitter v2 C. Angerer 10/2018/1 -> Mux9/1
  Torque Splitter v2 C. Angerer 10/2018/2 -> Mux9/2
  Torque Splitter v2 C. Angerer 10/2018/3 -> [n_Kupplung_geschlossen_VA]
  Torque Splitter v2 C. Angerer 10/2018/4 -> [p_v_TS_VA]
  [M_Rad_W_RF] -> Torque Splitter v2 C. Angerer 10/2018/3
  [M_Rad_W_LF] -> Torque Splitter v2 C. Angerer 10/2018/4
  [n_Rad_RF] -> Torque Splitter v2 C. Angerer 10/2018/1
  [n_Rad_LF] -> Torque Splitter v2 C. Angerer 10/2018/2
  [TS_HA] -> Drehzahlrückführung az HA/5(TS_HA)
  [n_Kupplung_geschlossen_HA] -> Drehzahlrückführung az HA/4(n_Kupplung_geschlossen_HA)
  Drehzahlrückführung az HA/1(n_motor) -> Simple E-Maschine HA/2
  [n_Kupplung_geschlossen_VA] -> Drehzahlrückführung az VA/4(n_Kupplung_geschlossen_VA)
  [TS_VA] -> Drehzahlrückführung az VA/5(TS_VA)
  Drehzahlrückführung az VA/1(n_motor) -> Simple E-Maschine VA/2
  [P_el_EM_rn_HA] -> Bus Creator4/4  "P_el_EM_rn_HA"
  Logical Operator/1 -> Add/1
  Discrete-Time Integrator6/1 -> kWs --> kWh6/1
  [pv_simEM_az_HA] -> Bus Creator3/2  "pv_simEM_az_HA"
  Bus Creator2/1 -> To Ws 5/1
  [pv_LE_HA_AZ] -> Discrete-Time Integrator14/1  "pv_LE_HA_AZ"
  [pv_OD_HA] -> Discrete-Time Integrator5/1  "pv_OD_HA"
  kWs --> kWh5/1 -> Bus Creator2/6  "Ev_OD_HA"
  Discrete-Time Integrator5/1 -> kWs --> kWh5/1
  kWs --> kWh3/1 -> Bus Creator2/4  "Ev_GTR_az_HA"
  kWs --> kWh14/1 -> Bus Creator2/15  "Ev_LE_HA_AZ"
  [pv_OD_HA] -> Bus Creator3/6  "pv_OD_HA"
  [pv_simEM_rn_HA] -> Bus Creator3/10  "pv_simEM_rn_HA"
  [pv_simEM_rn_HA] -> Discrete-Time Integrator9/1  "pv_simEM_rn_HA"
  [pv_LE_HA_AZ] -> Bus Creator3/15  "pv_LE_HA_AZ"
  [pv_GTR_az_HA] -> Bus Creator3/4  "pv_simGTR_az_HA"
  Discrete-Time Integrator11/1 -> kWs --> kWh11/1
  Discrete-Time Integrator/1 -> kWs --> kWh/1
  [pv_GTR_rn_HA] -> Bus Creator3/12  "pv_simGTR_rn_HA"
  [eta_LE_VA_RN] -> Bus Creator5/2  "eta_LE_VA_RN"
  Bus Creator4/1 -> To Ws 6/1  "P_el_EM"
  [p_v_TS_VA] -> Discrete-Time Integrator17/1  "PV_TS_VA"
  kWs --> kWh17/1 -> Bus Creator2/18
  Add21/1 -> Demux4/1
  Add/1 -> To Ws 7/1
  [eta_EM_rn_HA] -> Logical Operator45/1, Add33/2
  Add37/1 -> Demux12/1
  Add40/1 -> Demux13/1
  kWs --> kWh11/1 -> Bus Creator2/12  "Ev_GTR_rn_HA"
  [eta_LE_HA_AZ] -> Bus Creator5/3  "eta_LE_HA_AZ"
  Demux9/2 -> Product5/2, Add29/2  "P_LF"
  Demux8/1 -> RF/1  "LE_RF"
  [P_LE_DC_VA_AZ] -> Add43/1
  Logical Operator48/1 -> Add35/1
  [p_v_TS_VA] -> Bus Creator3/18
  [eta_OD_VA] -> Bus Creator1/1  "eta_OD_VA"
  LF1/1 -> Product11/1
  [P_el_EM_az_HA] -> Bus Creator4/3  "P_el_EM_az_HA"
  Bus Creator3/1 -> To Ws 1/1  "pv_ges"
  [eta_eUELG_HA] -> Add35/2, Logical Operator48/1
  Discrete-Time Integrator7/1 -> kWs --> kWh7/1
  Add36/1 -> Product8/2
  [eta_EM_az_HA] -> Logical Operator51/1, Add38/2
  Add29/1 -> Divide/2
  Logical Operator45/1 -> Add33/1
  Logical Operator6/1 -> Add7/1
  Logical Operator4/1 -> Add5/1
  Logical Operator1/1 -> Add2/1
  Bus Creator1/1 -> To Workspace20/1
  [eta_2GTR_az_HA] -> Logical Operator10/1, Add11/2
  Add13/1 -> HA/4
  Product1/1 -> Product2/1  "EM"
  Logical Operator52/1 -> Add39/1
  [eta_EM_rn_VA] -> Logical Operator35/1, Add21/2
  [eta_LE_VA_AZ] -> Bus Creator5/1  "eta_LE_VA_AZ"
  Logical Operator34/1 -> Add20/1
  Demux7/2 -> LF/3  "GTR_LF"
  Demux4/2 -> LF/2  "EM_LF"
  [P_el_EM_az_VA] -> Bus Creator4/1  "P_el_EM_az_VA"
  Demux4/1 -> RF/2  "EM_RF"
  Logical Operator11/1 -> Add12/1
  kWs --> kWh13/1 -> Bus Creator2/14  "Ev_LE_VA_RN"
  [eta_TS_VA] -> Add19/2, Logical Operator37/1
  [eta_OD_VA] -> Logical Operator36/1, Add22/2
  Logical Operator39/1 -> Add24/1
  Logical Operator36/1 -> Add22/1
  kWs --> kWh9/1 -> Bus Creator2/10  "Ev_EM_rn_HA"
  [eta_eUELG_VA] -> Add5/2, Logical Operator4/1
  Add27/1 -> Product1/1  "LE"
  Logical Operator2/1 -> Add3/1
  Add15/1 -> HA/5
  [eta_GTR_rn_HA] -> Add15/2, Logical Operator14/1
  [eta_2GTR_rn_VA] -> Add8/2, Logical Operator7/1
  Discrete-Time Integrator4/1 -> kWs --> kWh4/1
  Logical Operator3/1 -> Add4/1
  kWs --> kWh18/1 -> Bus Creator2/19
  [eta_2GTR_az_VA] -> Add3/2, Logical Operator2/1
  Add5/1 -> VA/4
  Add10/1 -> HA/1
  Add6/1 -> To Ws 8/1
  Add22/1 -> VA_diff/1
  [p_v_TS_HA] -> Bus Creator3/19
  Product9/1 -> Product12/2  "HA"
  [eta_LE_VA_AZ] -> Logical Operator42/1, Add27/2
  Add43/1 -> Product13/2, Add45/1  "P_VA"
  [eta_eUELG_VA] -> Add23/2, Logical Operator38/1
  RF1/1 -> Product10/1
  [pv_simEM_az_VA] -> Bus Creator3/1  "pv_simEM_az_VA"
  Demux14/2 -> Add43/3
  Logical Operator38/1 -> Add23/1
  [pv_ges_eUELG_HA] -> Bus Creator3/8  "pv_eUELG_HA"
  [pv_simEM_rn_VA] -> Bus Creator3/9  "pv_simEM_rn_VA"
  VA/1 -> [eta_VA]
  [eta_OD_HA] -> Logical Operator46/1, Add34/2
  [eta_OD_VA] -> Logical Operator3/1, Add4/2
  [pv_OD_VA] -> Bus Creator3/5  "pv_OD_VA"
  Divide2/1 -> To Ws 12/1  "eta_AS_ges"
  Logical Operator12/1 -> Add13/1
  Add45/1 -> Divide2/2  "P_ges"
  [eta_EM_rn_VA] -> Logical Operator5/1, Add6/2
  [eta_EM_az_HA] -> Add9/2, Logical Operator8/1
  Discrete-Time Integrator12/1 -> kWs --> kWh12/1
  Add46/1 -> Divide2/1
  Product8/1 -> Product9/1  "GTR"
  Discrete-Time Integrator1/1 -> kWs --> kWh1/1
  Add16/1 -> HA/6
  Demux15/2 -> Add44/3
  Product10/1 -> Add42/1
  Add26/1 -> Product1/2
  Product12/1 -> To Ws 4/1, Product14/2  "eta_HA"
  Demux9/1 -> Add29/1, Product4/2  "P_RF"
  Bus Creator5/1 -> To Ws 11/1
  [eta_GTR_rn_VA] -> Logical Operator34/1, Add20/2
  Product14/1 -> Add46/2
  [pv_GTR_rn_VA] -> Bus Creator3/11  "pv_simGTR_rn_VA"
  [pv_ges_eUELG_VA] -> Discrete-Time Integrator6/1  "pv_eUELG_VA"
  Add35/1 -> HA_diff1/2
  [pv_GTR_rn_HA] -> Discrete-Time Integrator11/1  "pv_simGTR_rn_HA"
  [eta_GTR_az_HA] -> Logical Operator49/1, Add36/2
  Add14/1 -> To Ws 10/1
  Discrete-Time Integrator14/1 -> kWs --> kWh14/1
  VA_diff/1 -> Product3/2
  Demux10/1 -> RF1/2  "EM_RF"
  Product2/1 -> Product3/1  "GTR"
  [eta_OD_HA] -> Bus Creator1/2  "eta_OD_HA"
  [pv_GTR_az_VA] -> Discrete-Time Integrator2/1  "pv_simGTR_az_VA"
  [pv_GTR_az_HA] -> Discrete-Time Integrator3/1  "pv_simGTR_az_HA"
  [eta_EM_az_VA] -> Logical Operator41/1, Add26/2
  Demux15/1 -> Add44/2
  [pv_ges_eUELG_HA] -> Discrete-Time Integrator7/1  "pv_eUELG_HA"
  Add1/1 -> HA/7
  kWs --> kWh1/1 -> Bus Creator2/2  "Ev_EM_az_HA"
  Discrete-Time Integrator2/1 -> kWs --> kWh2/1
  Logical Operator50/1 -> Add37/1
  [eta_LE_HA_AZ] -> Logical Operator52/1, Add39/2
  kWs --> kWh10/1 -> Bus Creator2/11  "Ev_GTR_rn_VA"
  Logical Operator37/1 -> Add19/1
  Demux11/1 -> RF1/3  "GTR_RF"
  Add39/1 -> Product7/1  "LE"
  Discrete-Time Integrator3/1 -> kWs --> kWh3/1
  [P_LE_DC_HA_RN] -> Demux15/1
  Demux7/1 -> RF/3  "GTR_RF"
  RF/1 -> Product4/1
  Demux14/1 -> Add43/2
  Discrete-Time Integrator17/1 -> kWs --> kWh17/1
  Logical Operator15/1 -> Add16/1
  Logical Operator49/1 -> Add36/1
  Logical Operator9/1 -> Add10/1
  Discrete-Time Integrator8/1 -> kWs --> kWh8/1
  [eta_LE_HA_RN] -> Bus Creator5/4  "eta_LE_HA_RN"
  kWs --> kWh15/1 -> Bus Creator2/16  "Ev_LE_HA_RN"
  [P_Batt] -> Bus Creator4/6  "pv_LE_VA_RN"
  Add20/1 -> Demux7/1
  [pv_GTR_rn_VA] -> Discrete-Time Integrator10/1  "pv_simGTR_rn_VA"
  Product11/1 -> Add42/2
  Add33/1 -> Demux10/1
  Logical Operator40/1 -> Add25/1
  Add32/1 -> Demux11/1
  Add34/1 -> HA_diff1/1
  Add38/1 -> Product7/2
  Logical Operator14/1 -> Add15/1
  Divide/1 -> Product6/1
  Add31/1 -> HA_diff1/3
  Logical Operator5/1 -> Add6/1
  [pv_simEM_az_HA] -> Discrete-Time Integrator1/1  "pv_simEM_az_HA"
  [pv_GTR_az_VA] -> Bus Creator3/3  "pv_simGTR_az_VA"
  Demux12/2 -> LF1/1  "LE_LF"
  Demux13/2 -> Product11/2, Add41/2  "P_LF"
  kWs --> kWh6/1 -> Bus Creator2/7  "Ev_eUELG_VA"
  [eta_TS_HA] -> Add31/2, Logical Operator47/1
  Add41/1 -> Divide1/2
  Demux13/1 -> Add41/1, Product10/2  "P_RF"
  Product6/1 -> To Ws 3/1, Product13/1  "eta_VA"
  Add42/1 -> Divide1/1
  Logical Operator46/1 -> Add34/1
  [P_LE_DC_HA_AZ] -> Add44/1
  [pv_LE_VA_RN] -> Bus Creator3/14  "pv_LE_VA_RN"
  Discrete-Time Integrator13/1 -> kWs --> kWh13/1
  [eta_TS_VA] -> Add18/2, Logical Operator33/1
  Add9/1 -> To Ws 9/1
  Add18/1 -> VA/7
  [eta_TS_HA] -> Add1/2, Logical Operator32/1
  [eta_LE_HA_RN] -> Add37/2, Logical Operator50/1
  Logical Operator32/1 -> Add1/1
  Add3/1 -> VA/2
  kWs --> kWh2/1 -> Bus Creator2/3  "Ev_GTR_az_VA"
  [P_LE_DC] -> Bus Creator4/5  "pv_LE_VA_AZ"
  [p_v_TS_HA] -> Discrete-Time Integrator18/1  "PV_TS_HA"
  Discrete-Time Integrator18/1 -> kWs --> kWh18/1
  Add11/1 -> HA/2
  Logical Operator44/1 -> Add32/1
  Add12/1 -> HA/3
  [eta_2GTR_rn_HA] -> Logical Operator15/1, Add16/2
  [P_LE_DC_VA_RN] -> Demux14/1
  Discrete-Time Integrator15/1 -> kWs --> kWh15/1
  [eta_EM_rn_HA] -> Add14/2, Logical Operator13/1
  Add4/1 -> VA/3
  Add8/1 -> VA/6
  Logical Operator8/1 -> Add9/1
  [eta_eUELG_HA] -> Logical Operator12/1, Add13/2
  Discrete-Time Integrator10/1 -> kWs --> kWh10/1
  [eta_OD_HA] -> Add12/2, Logical Operator11/1
  Add2/1 -> VA/1
  [pv_simEM_az_VA] -> Discrete-Time Integrator/1  "pv_simEM_az_VA"
  [eta_GTR_az_HA] -> Logical Operator9/1, Add10/2
  [pv_LE_VA_RN] -> Discrete-Time Integrator13/1  "pv_LE_VA_RN"
  Logical Operator41/1 -> Add26/1
  Logical Operator42/1 -> Add27/1
  Add24/1 -> Product2/2
  [pv_LE_VA_AZ] -> Bus Creator3/13  "pv_LE_VA_AZ"
  Add7/1 -> VA/5
  Logical Operator47/1 -> Add31/1
  Demux12/1 -> RF1/1  "LE_RF"
  Demux10/2 -> LF1/2  "EM_LF"
  Demux11/2 -> LF1/3  "GTR_LF"
  Add30/1 -> Divide/1
  [pv_Batt] -> Discrete-Time Integrator16/1  "pv_Batt"
  Product4/1 -> Add30/1
  [eta_EM_az_VA] -> Logical Operator/1, Add/2
  [pv_LE_HA_RN] -> Discrete-Time Integrator15/1  "pv_LE_HA_RN"
  Add23/1 -> VA_diff/2
  Logical Operator51/1 -> Add38/1
  Logical Operator33/1 -> Add18/1
  [P_LE_DC_VA_RN] -> Logical Operator43/1, Add28/2
  Divide1/1 -> Product12/1
  Product13/1 -> Add46/1
  Product5/1 -> Add30/2
  Add44/1 -> Add45/2, Product14/1  "P_HA"
  kWs --> kWh8/1 -> Bus Creator2/9  "Ev_EM_rn_VA"
  Add28/1 -> Demux9/1
  Logical Operator43/1 -> Add28/1
  kWs --> kWh7/1 -> Bus Creator2/8  "Ev_eUELG_HA"
  kWs --> kWh/1 -> Bus Creator2/1  "Ev_EM_az_VA"
  [pv_simEM_rn_VA] -> Discrete-Time Integrator8/1  "pv_simEM_rn_VA"
  Product7/1 -> Product8/1  "EM"
  Demux8/2 -> LF/1  "LE_LF"
  Add19/1 -> VA_diff/3
  [P_el_EM_rn_VA] -> Bus Creator4/2  "P_el_EM_rn_VA"
  [pv_ges_eUELG_VA] -> Bus Creator3/7  "pv_eUELG_VA"
  Logical Operator53/1 -> Add40/1
  [eta_LE_VA_RN] -> Add25/2, Logical Operator40/1
  LF/1 -> Product5/1
  [eta_GTR_rn_HA] -> Logical Operator44/1, Add32/2
  [eta_GTR_az_VA] -> Logical Operator1/1, Add2/2
  [pv_Batt] -> Bus Creator3/17  "pv_Batt"
  HA_diff1/1 -> Product9/2
  Discrete-Time Integrator9/1 -> kWs --> kWh9/1
  Logical Operator13/1 -> Add14/1
  Logical Operator35/1 -> Add21/1
  Product3/1 -> Product6/2  "VA"
  [eta_GTR_az_VA] -> Logical Operator39/1, Add24/2
  [P_LE_DC_HA_RN] -> Logical Operator53/1, Add40/2
  Logical Operator7/1 -> Add8/1
  kWs --> kWh12/1 -> Bus Creator2/13  "Ev_LE_VA_AZ"
  Discrete-Time Integrator16/1 -> kWs --> kWh16/1
  Logical Operator10/1 -> Add11/1
  [pv_LE_HA_RN] -> Bus Creator3/16  "pv_LE_HA_RN"
  [pv_OD_VA] -> Discrete-Time Integrator4/1  "pv_OD_VA"
  HA/1 -> [eta_HA]
  Add25/1 -> Demux8/1
  kWs --> kWh4/1 -> Bus Creator2/5  "Ev_OD_VA"
  [pv_LE_VA_AZ] -> Discrete-Time Integrator12/1  "pv_LE_VA_AZ"
  [eta_GTR_rn_VA] -> Logical Operator6/1, Add7/2
  kWs --> kWh16/1 -> Bus Creator2/17  "Ev_Batt"
  Simple E-Maschine VA/2 -> Mehrstufiges und mehrgängiges Getriebe az/2, [n_mot_az_va]  "1"
  Drehzahlrückführung rn VA fuer mmG/1 -> Simple E-Maschine radnah/2, Mehrstufiges und mehrgängiges Getriebe rn/2, [n_mot_rn_va]
  MATLAB Function4/1(RIX) -> [RIX_HA_Delayed]
  MATLAB Function2/1(RIX) -> [RIX_VA_Delayed]
  Simple E-Maschine radnah1/1 -> MATLAB Function5/1(u), Mehrstufiges und mehrgängiges Getriebe rn1/1, [m_mot_rn_ha]  "2"
  Simple E-Maschine HA/1 -> [m_mot_az_ha], MATLAB Function4/1(u), Mehrstufiges und mehrgängiges Getriebe az1/1  "1"
  Simple E-Maschine radnah/1 -> MATLAB Function3/1(u), Mehrstufiges und mehrgängiges Getriebe rn/1, [m_mot_rn_va]  "2"
  Simple E-Maschine VA/1 -> MATLAB Function2/1(u), [m_mot_az_va], Mehrstufiges und mehrgängiges Getriebe az/1  "1"
  [RIX_HA_Delayed] -> Offenes Differential HA/4
  [RIX_VA_Delayed] -> Torque Splitter v2 C. Angerer 10/2018/6
  MATLAB Function5/1(RIX) -> Mehrstufiges und mehrgängiges Getriebe rn1/5
  [P_Batt_eUELG_HA] -> Add17/8
  [P_Batt_eUELG_VA] -> Add17/7
  [TS_VA] -> Torque Splitter v2 C. Angerer 10/2018/Enable
  [eTV_VA] -> Elektrisches Überlagerungsgetriebe VA/Enable
  Mux7/1 -> Multiport Switch2/5
  Mux1/1 -> Momentenrückführung HA fuer mmG/1, Keine Rückführung1/1, MATLAB Function1/1(u)

== system ZSM_TeslaModelS_statKreisfahrt/Vehicle/Betriebsstrategie ==
  FromDriver : Inport
  FromFahrzeugmodell : Inport  Port=2
  FromEnvironment : Inport  Port=3
  10 Hz Tiefpass : Subsystem
  Bus Creator : BusCreator  Inputs=3
  Bus Selector : BusSelector  OutputSignals=M_wheel
  Bus Selector1 : BusSelector  OutputSignals=delta_wheel
  Bus Selector2 : BusSelector  OutputSignals=ENV_road_mu
  Momentenverteilung_und_Schaltstrategie1 : Subsystem
  sv_BetriebsstrategieOut : ToWorkspace  Commented=on  VariableName=sv_BetriebsstrategieOut  SaveFormat=Timeseries  SampleTime=-1
      settings: Decimation=savedec
  BetriebsstrategieOut : Outport  VectorParamsAs1DForOutWhenUnconnected=off
  wires:
  FromFahrzeugmodell/1 -> Momentenverteilung_und_Schaltstrategie1/3(input), Bus Selector1/1
  Momentenverteilung_und_Schaltstrategie1/1(M_antr) -> 10 Hz Tiefpass/1(In1)  "M_antr"
  Bus Creator/1 -> BetriebsstrategieOut/1, sv_BetriebsstrategieOut/1
  FromDriver/1 -> Bus Selector/1
  Bus Selector/1 -> Momentenverteilung_und_Schaltstrategie1/1(M_wheel)  "<M_wheel>"
  Momentenverteilung_und_Schaltstrategie1/2(M_brems) -> Bus Creator/2  "M_brems"
  Bus Selector1/1 -> Momentenverteilung_und_Schaltstrategie1/2(delta_wheel)  "<delta_wheel>"
  Momentenverteilung_und_Schaltstrategie1/3(Schaltstrategie) -> Bus Creator/3  "Schaltstrategie"
  Bus Selector2/1 -> Momentenverteilung_und_Schaltstrategie1/4(mu_road)  "<ENV_road_mu>"
  FromEnvironment/1 -> Bus Selector2/1
  10 Hz Tiefpass/1(Out1) -> Bus Creator/1
